simulink model "Model_plane1_new"  (R2024a)
settings: Solver=FixedStepAuto  StartTime=0  StopTime=2000  FixedStep=1  RelTol=1e-3
model workspace (MAT data in the model file):
  Alfa = [-2 4 10 16]
  Alfa_RUD = 0.55
  Alfa_table = [-4 0 5 10 20]
  Alfa_y = [-4 6 8 9 10 12 14]
  Cxa_table = [0.03434  0.0358  0.04274; 0.02598  0.0252  0.0262; 0.04151  0.0505  0.0883; 0.122  0.1649  0.2341; 0.502  0.538  0.666]
  Cy_DB = [0.01242 0.01286 0.01457]
  Cy_fi = [0.00623 0.00643 0.00626]
  Cya = [-0.276  -0.33  -0.39; 0.859  0.991  0.82; 1.085  1.211  1.1; 1.2  1.275  1.031; 1.296  1.29  1.018; 1.45  1.178  1.043; 1.461  1.163  1.081]
  Del_B = -5
  H = [339 3256 4060 8000 12000]
  H_table = [0 2000 4000 6000 8000 10000]
  I = [1000 1000 4500000]
  K_H = -0.3
  K_p = 0.3
  K_w = 1.5
  M_C = [0.4 0.6 0.82]
  M_mz = [0.2 0.4 0.6 0.8]
  M_mz2 = [0.4 0.7 0.85]
  M_table = [0.4 0.7 0.82]
  M_y = [0.4 0.7 0.82]
  P = [50000 40000 32000 25600 20480]
  Psi0 = 0
  Skr = 131
  Teta0 = 0
  V0 = 135
  a_table = [340.3 339.5 338.8 338 337.2 336.4]
  ba = 3.466
  fi = 0
  fi_P = 2
  g = 9.81
  lz = 4500000
  mla = 60000
  mz_DB = [-0.035 -0.0358 -0.037 -0.0377]
  mz_alfa = [-0.0282 -0.0282 -0.0289 -0.0404]
  mz_alfa2 = [-8.163  -8.762  -9.714; -8.163  -8.762  -9.583; -7.975  -7.991  -7.868; -6.514  -6.413  -6.732]
  mz_fi = [-0.0695 -0.0714 -0.0739 -0.0832]
  mz_omz = [-23.768  -25.3  -28.284; -23.768  -25.3  -27.903; -23.222  -22.6  -23.32; -18.967  -18.52  -19.601]
  n_dvig = 2
  out = Simulink.SimulationOutput
  out.Data.tout = [0 1.67688873362e-06 9.33181354111e-06 4.76064375786e-05 0.000238979557766 0.0011958451587 0.00598017316339 0.0291858115735 0.107609227908 0.294605508218 0.534390352194 0.619831316604 ... (6422 elements, 6422x1)]
  out.Metadata = Simulink.SimulationMetadata
  out.Metadata.ModelInfo.ModelName = 'Model_plane2'
  out.Metadata.ModelInfo.ModelVersion = '1.11'
  out.Metadata.ModelInfo.ModelFilePath = 'C:\Users\Анастасия\Универ\Mathlab\Модель самолёта\Model_plane2.slx'
  out.Metadata.ModelInfo.UserID = 'Анастасия'
  out.Metadata.ModelInfo.MachineName = 'DESKTOP-OE36224'
  out.Metadata.ModelInfo.Platform = 'PCWIN64'
  out.Metadata.ModelInfo.ModelStructuralChecksum = [329193822; 1830100004; 2373400892; 4162968501]
  out.Metadata.ModelInfo.SimulationMode = 'normal'
  out.Metadata.ModelInfo.StartTime = 0
  out.Metadata.ModelInfo.StopTime = 100
  out.Metadata.ModelInfo.SolverInfo.Type = 'Variable-Step'
  out.Metadata.ModelInfo.SolverInfo.Solver = 'ode45'
  out.Metadata.ModelInfo.SolverInfo.MaxStepSize = 2
  out.Metadata.ModelInfo.SimulinkVersion.Name = 'Simulink'
  out.Metadata.ModelInfo.SimulinkVersion.Version = '24.1'
  out.Metadata.ModelInfo.SimulinkVersion.Release = '(R2024a)'
  out.Metadata.ModelInfo.SimulinkVersion.Date = '19-Nov-2023'
  out.Metadata.ModelInfo.LoggingInfo.LoggingToFile = 'off'
  out.Metadata.TimingInfo.WallClockTimestampStart = '2025-02-14 11:01:22'
  out.Metadata.TimingInfo.WallClockTimestampStop = '2025-02-14 11:01:24'
  out.Metadata.TimingInfo.InitializationElapsedWallTime = 1.1990057
  out.Metadata.TimingInfo.ExecutionElapsedWallTime = 1.0786509
  out.Metadata.TimingInfo.TerminationElapsedWallTime = 0.0112241
  out.Metadata.TimingInfo.TotalElapsedWallTime = 2.2888807
  out.Metadata.TimingInfo.ProfilerData = 'Profiler is not enabled'
  out.Metadata.ExecutionInfo.StopEvent = 'ReachedStopTime'
  out.Metadata.ExecutionInfo.StopEventSource = []
  out.Metadata.ExecutionInfo.StopEventDescription = 'Reached stop time of 100'
  out.Metadata.ExecutionInfo.ErrorDiagnostic = []
  out.Metadata.ExecutionInfo.WarningDiagnostics.Diagnostic = MSLDiagnostic
  out.Metadata.ExecutionInfo.WarningDiagnostics.Diagnostic.identifier = 'Simulink:blocks:DivideByZero'
  out.Metadata.ExecutionInfo.WarningDiagnostics.Diagnostic.message = 'Division by zero in ''<a href="matlab:open_and_hilite_hyperlink (''Model_plane2/Уравнения продольного движения в связанной системе координат/Блок расчёта угла атаки Alfa/Divide'',''error'')">Model_plane2/Уравнения продольного движения в связанной системе координат/Блок расчёта угла атаки Alfa/Divide</a>'''
  out.Metadata.ExecutionInfo.WarningDiagnostics.Diagnostic.paths = {'Model_plane2/Уравнения продольного движения в связанной системе координат/Блок расчёта угла атаки Alfa/Divide'}
  out.Metadata.ExecutionInfo.WarningDiagnostics.Diagnostic.arguments = {'Model_plane2/Уравнения продольного движения в связанной системе координат/Блок расчёта угла атаки Alfa/Divide'}
  out.Metadata.ExecutionInfo.WarningDiagnostics.Diagnostic.stack = struct([])
  out.Metadata.ExecutionInfo.WarningDiagnostics.Diagnostic.actionProp = '22 serialization::archive 19 0 0 0  0 1 0 0 1 1 0 0 0 0 0 1 47 SL_SERVICES:utils:EMBEDDED____ACTION____WRAPPER 2 2 0 0 183 0 109 97 116 108 97 98 58 83 105 109 117 108 105 110 107 46 83 117 112 112 114 101 115 115 101 100 68 105 97 103 110 111 115 116 105 99 40 123 39 77 111 100 101 108 95 112 108 97 110 101 50 47 1059 1088 1072 1074 1085 1077 1085 1080 1103 32 1087 1088 1086 1076 1086 1083 1100 1085 1086 1075 1086 32 1076 1074 1080 1078 1077 1085 1080 1103 32 1074 32 1089 1074 1103 1079 1072 1085 1085 1086 1081 32 1089 1080 1089 1090 1077 1084 1077 32 1082 1086 1086 1088 1076 1080 1085 1072 1090 47 1041 1083 1086 1082 32 1088 1072 1089 1095 1105 1090 1072 32 1091 1075 1083 1072 32 1072 1090 1072 1082 1080 32 65 108 102 97 47 68 105 118 105 100 101 39 125 44 39 83 105 109 117 108 105 110 107 58 98 108 111 99 107 115 58 68 105 118 105 100 101 66 121 90 101 114 111 39 41 59 2 0 0 1 6 0 0 0 0 0  1 0 0 0 0'
  out.Metadata.ExecutionInfo.WarningDiagnostics.Diagnostic.metaDataProp.UI = []
  out.Metadata.ExecutionInfo.WarningDiagnostics.Diagnostic.metaDataProp.STAGE = []
  out.Metadata.ExecutionInfo.WarningDiagnostics.Diagnostic.metaDataProp.CATEGORY = []
  out.Metadata.ExecutionInfo.WarningDiagnostics.Diagnostic.metaDataProp.COMPONENT = []
  out.Metadata.ExecutionInfo.WarningDiagnostics.Diagnostic.metaDataProp.MDL_NAME = []
  out.Metadata.ExecutionInfo.WarningDiagnostics.Diagnostic.metaDataProp.ACTION = '22 serialization::archive 19 0 0 0  0 1 0 0 1 1 0 0 0 0 0 1 47 SL_SERVICES:utils:EMBEDDED____ACTION____WRAPPER 2 2 0 0 183 0 109 97 116 108 97 98 58 83 105 109 117 108 105 110 107 46 83 117 112 112 114 101 115 115 101 100 68 105 97 103 110 111 115 116 105 99 40 123 39 77 111 100 101 108 95 112 108 97 110 101 50 47 1059 1088 1072 1074 1085 1077 1085 1080 1103 32 1087 1088 1086 1076 1086 1083 1100 1085 1086 1075 1086 32 1076 1074 1080 1078 1077 1085 1080 1103 32 1074 32 1089 1074 1103 1079 1072 1085 1085 1086 1081 32 1089 1080 1089 1090 1077 1084 1077 32 1082 1086 1086 1088 1076 1080 1085 1072 1090 47 1041 1083 1086 1082 32 1088 1072 1089 1095 1105 1090 1072 32 1091 1075 1083 1072 32 1072 1090 1072 1082 1080 32 65 108 102 97 47 68 105 118 105 100 101 39 125 44 39 83 105 109 117 108 105 110 107 58 98 108 111 99 107 115 58 68 105 118 105 100 101 66 121 90 101 114 111 39 41 59 2 0 0 1 6 0 0 0 0 0  1 0 0 0 0'
  out.Metadata.ExecutionInfo.WarningDiagnostics.Diagnostic.metaDataProp.DOC = []
  out.Metadata.ExecutionInfo.WarningDiagnostics.Diagnostic.metaDataProp.SUB_CATEGORY = []
  out.Metadata.ExecutionInfo.WarningDiagnostics.Diagnostic.metaDataProp.MSTACK_PRESERVE = []
  out.Metadata.ExecutionInfo.WarningDiagnostics.Diagnostic.metaDataProp.DOUBLE_ARGS = []
  out.Metadata.ExecutionInfo.WarningDiagnostics.Diagnostic.metaDataProp.USER_DATA = []
  out.Metadata.ExecutionInfo.WarningDiagnostics.Diagnostic.priority = 2
  out.Metadata.ExecutionInfo.WarningDiagnostics.SimulationPhase = 'Execution'
  out.Metadata.ExecutionInfo.WarningDiagnostics.SimulationTime = 0
  out.Metadata.AppInfo = struct()
  pitch = 1
  pitch0 = 0
  q_table = [1.225 1.0065 0.8194 0.6601 0.5258 0.4135]
  roll0 = 0
  wx0 = 0
  wy0 = 0
  wz0 = 0
  x0 = 0
  xy = [240000 6200]
  y0 = 5000
  yaw0 = 0
  z0 = 0
settings Model: Creator=Анастасия  LastModifiedBy=Анастасия
settings SolverCC: MaxConsecutiveMinStep=5
settings DebuggingCC: UnderSpecifiedDimensionMsg=warning

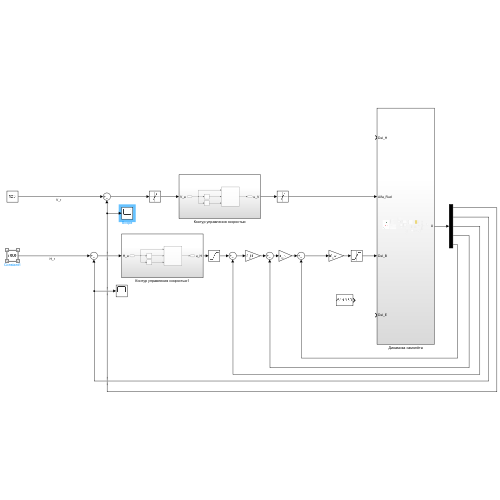
[thumbnail: Simulink's stored preview of the top-level diagram]
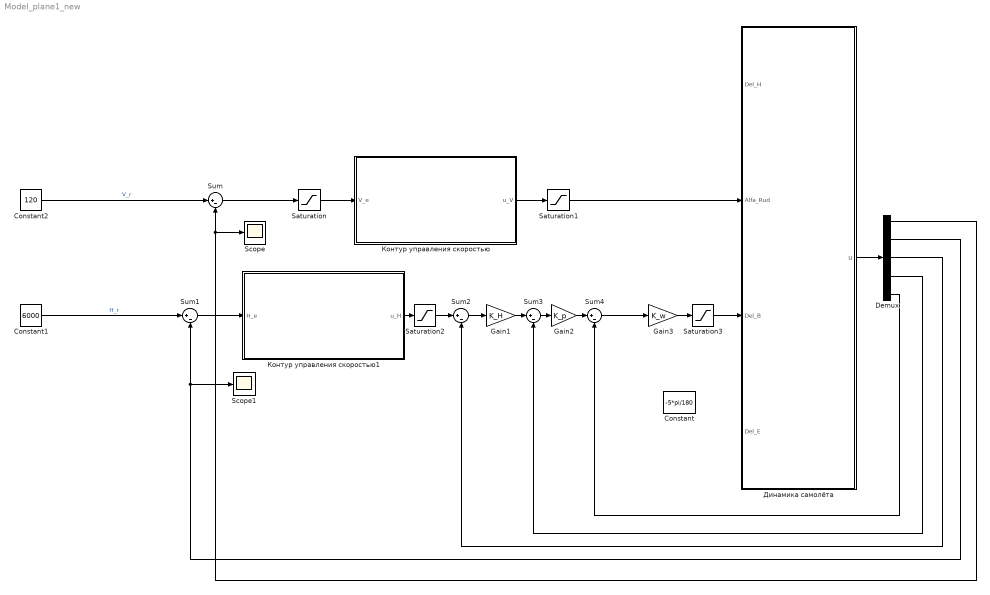
== system Model_plane1_new ==
  Constant : Constant  Value=-5*pi/180
  Constant1 : Constant  Value=6000
  Constant2 : Constant  Value=120
  Demux : Demux  Outputs=5
  Gain1 : Gain  Gain=K_H
  Gain2 : Gain  Gain=K_p
  Gain3 : Gain  Gain=K_w
  Saturation : Saturate  UpperLimit=300  LowerLimit=-300
  Saturation1 : Saturate  UpperLimit=300  LowerLimit=0
  Saturation2 : Saturate  UpperLimit=10  LowerLimit=-10
  Saturation3 : Saturate  UpperLimit=25*pi/180  LowerLimit=-35*pi/180
  Scope : Scope
  Scope1 : Scope
  Sum{,1..4} (5 alike) : Sum  Inputs=|+-
  Динамика самолёта : Subsystem
  Контур управления скоростью : Subsystem
  Контур управления скоростью1 : Subsystem
  wires:
  Constant2/1 -> Sum/1  "V_r"
  Sum/1 -> Saturation/1
  Saturation/1 -> Контур управления скоростью/1(V_e)
  Контур управления скоростью/1(u_V) -> Saturation1/1
  Динамика самолёта/1(U) -> Demux/1
  Demux/1 -> Scope/1, Sum/2
  Constant1/1 -> Sum1/1  "H_r"
  Demux/2 -> Scope1/1, Sum1/2
  Sum1/1 -> Контур управления скоростью1/1(H_e)
  Контур управления скоростью1/1(u_H) -> Saturation2/1
  Saturation2/1 -> Sum2/1
  Sum2/1 -> Gain1/1
  Gain1/1 -> Sum3/1
  Sum3/1 -> Gain2/1
  Gain2/1 -> Sum4/1
  Sum4/1 -> Gain3/1
  Gain3/1 -> Saturation3/1
  Demux/3 -> Sum2/2
  Demux/4 -> Sum3/2
  Demux/5 -> Sum4/2
  Saturation1/1 -> Динамика самолёта/2(Alfa_Rud)
  Saturation3/1 -> Динамика самолёта/3(Del_B)

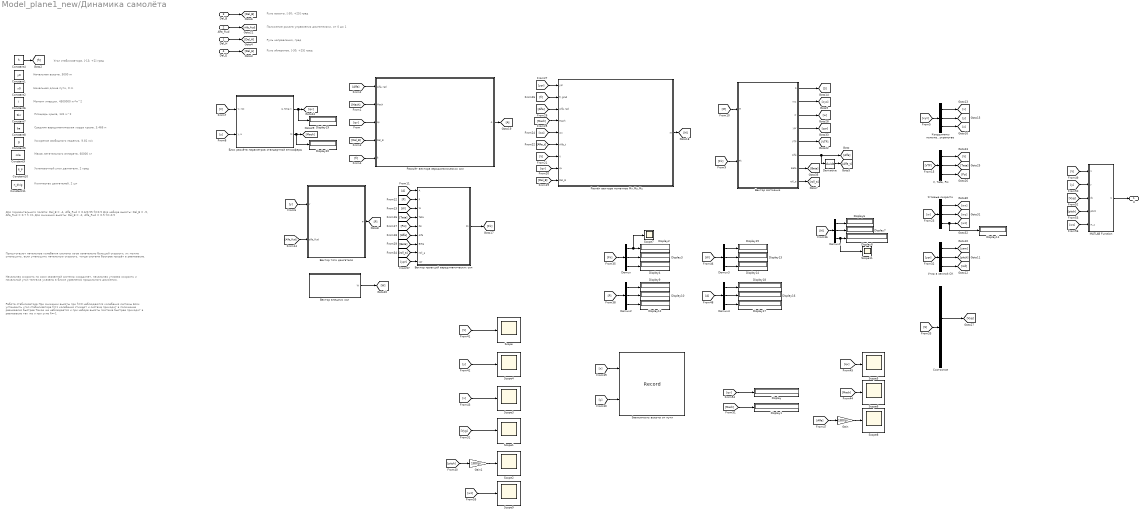
== system Model_plane1_new/Динамика самолёта ==
  note: Руль высоты, [-30; +25] град
  note: Начальная скорость по осям связанной системы координат, начальная угловая скорость и начальный угол тангажа указаны в блоке уравнения продольного движения.
  note: Количество двигателей, 2 шт
  note: Присутствуют начальные колебания системы из-за изначально большой скорости, их можно уменьшить, если уменьшить начальную скорость, тогда система быстрее придёт в равновесие.
  note: Установочный угол двигателя, 2 град
  note: Ускорение свободного падения, 9.81 м/c
  note: Масса летательного аппарата, 60000 кг
  note: Положение рычага управления двигателями, от 0 до 1
  note: Для горизонтального полёта:
      | Del_B = -4, Alfa_Rud = 0.6/0.55 fi=0.5
      | Для набора высоты:
      | Del_B = -5, Alfa_Rud = 0.7 fi =1
      | Для снижения высоты:
      | Del_B = -2, Alfa_Rud = 0.5 fi=-0.5
  note: Начальная длина пути, 0 m
  note: Работа стабилизатора
      | При снижении высоты при fi=0 наблюдаются колебания системы
      | Если установить угол стабилизатора fi=1 колебания стихают и систама приходит в положение равновесия быстрее
      | Такое же наблюдается и при наборе высоты (система быстрее приходит в равновесие так же и при угле fi=-1
  note: Средняя аэродинамическая хорда крыла, 3.466 м
  note: Площадь крыла, 131 м^2
  note: Начальная высота, 5000 m
  note: Момент инерции, 4500000 кг*м^2
  note: Угол стабилизатора, [-13; +2] град
  note: Руль направления, град
  note: Руль эйлеронов, [-30; +25] град
  Del_H : Inport
  Alfa_Rud : Inport  Port=2
  Del_B : Inport  Port=3
  Del_E : Inport  Port=4
  Constant1 : Constant  Value=y0
  Constant10 : Constant  Value=fi_P
  Constant11 : Constant  Value=n_dvig
  Constant2 : Constant  Value=x0
  Constant4 : Constant  Value=fi
  Constant5 : Constant  Value=g
  Constant6 : Constant  Value=I
  Constant7 : Constant  Value=Skr
  Constant8 : Constant  Value=ba
  Constant9 : Constant  Value=mla
  Demux{,1..4} (5 alike) : Demux  Outputs=3
  Derivative : Derivative
  Display{,1..4,6..20} (20 alike) : Display
  From11 : From
  From48 : From
  Gain : Gain  Gain=180/pi
  Gain1 : Gain  Gain=180/pi
  Goto19 : Goto
  MATLAB Function : MATLAB Function  TreatAsAtomicUnit=on
  Scope{,1..9,11} (11 alike) : Scope
  "V, Teta, Psi" : Demux  Outputs=3
  Блок расчёта параметров стандартной атмосферы : Subsystem
  Вектор внешних сил : Subsystem
  Вектор проекций аэродинамических сил : Subsystem
  Вектор состояния : Subsystem
  Вектор тяги двигателя : Subsystem
  Зависимость высоты от пути : Record  FileSettingsInternal="{\"entries\":[{\"content\":{\"excelSettings\":{\"content\":{},\"type\":\"Streamout.ExcelSettings\"}},\"type\":\"Streamout.FileSettingStorage\",\"uuid\":\"\"}],\"packageUris\":[\"http:\\/\\/schema.mathworks.com\\/mf0\\/streamout_blocks\\/R2020a\"],\"version\":\"1.0\"}"  Layout=[1 1]  SignalsInternal="{\"entries\":[{\"content\":{\"signals\":[{\"content\":{\"blockPath\":[],\"dimensions\":[1],\"domain\":\"\",\"lineColor\":\"#a2142f\",\"plots\":[ 1 ],\"port\":1,\"sid\":[\"\"],\"signalID\":1,\"signalName\":\"From39\"},\"type\":\"RecordBlkView.Signal\",\"uuid\":\"\"},{\"content\":{\"blockPath\":[],\"dimensions\":[1],\"domain\":\"\",\"lineColor\":\"#139fff\",\"plots\":[ 1 ],\"port\":2,\"sid\":[\"\"],\"signalID\":2,\"signalName\":\"From30\"},\"type\":\"RecordBlkView.Signal\",\"uuid\":\"\"}]},\"type\":\"RecordBlkView.InputSignals\",\"uuid\":\"\"}],\"packageUris\":[\"http:\\/\\/schema.mathworks.com\\/mf0\\/streamout_blocks\\/R2020a\"],\"version\":\"1.0\"}"  VisualizationBindings="{\"xyplotplugin\":{\"info\":[{\"series\":[{\"bindingParametersList\":[{\"parameter\":\"X-Axis\",\"signalID\":1,\"signalName\":\"From39\"},{\"parameter\":\"Y-Axis\",\"signalID\":2,\"signalName\":\"From30\"}],\"seriesID\":0}],\"subplotID\":1}]}}"  CompatibilityTag=XY  st=-1
  Координаты положения в пространстве : Demux  Outputs=3
  Рассчёт вектора аэродинамических сил : Subsystem
  Расчёт вектора мометнов Mx,My,Mz : Subsystem
  Состояние : Demux  Outputs=12
  Угловые скорости : Demux  Outputs=3
  Углы в земной СК : Demux  Outputs=3
  U : Outport
  wires:
  Constant4/1 -> [fi]
  [V] -> Блок расчёта параметров стандартной атмосферы/1("V, м/с")
  [y] -> Блок расчёта параметров стандартной атмосферы/2("y, м")
  Блок расчёта параметров стандартной атмосферы/2(М) -> Display20/1, [Mach]
  Блок расчёта параметров стандартной атмосферы/1("q, Н/кв.м") -> Display19/1, [qv]
  Вектор состояния/6(Alfa) -> Derivative/1, [Alfa]
  Derivative/1 -> [Alfa_t]
  [qv] -> Рассчёт вектора аэродинамических сил/3(qv)
  [Mach] -> Рассчёт вектора аэродинамических сил/2(Mach)
  [Alfa] -> Рассчёт вектора аэродинамических сил/1("Alfa, rad")
  [Del_B] -> Рассчёт вектора аэродинамических сил/4(Del_B)
  Del_B/1 -> [Del_B]
  [fi] -> Рассчёт вектора аэродинамических сил/5(fi)
  Вектор тяги двигателя/1(P) -> [P]
  Вектор состояния/2(xyz) -> [xyz]
  [xyz] -> Координаты положения в пространстве/1
  Координаты положения в пространстве/1 -> [x]
  Координаты положения в пространстве/2 -> [y]
  Координаты положения в пространстве/3 -> [z]
  [y] -> Вектор тяги двигателя/1(y)
  Вектор проекций аэродинамических сил/1(Fk) -> [Fk]
  [Fk] -> Вектор состояния/2(Fk)
  Расчёт вектора мометнов Mx,My,Mz/1(M) -> [M]
  Рассчёт вектора аэродинамических сил/1(A) -> Goto19/1
  From11/1 -> Вектор проекций аэродинамических сил/1(A)
  Вектор внешних сил/1(W) -> [W]
  [P] -> Вектор проекций аэродинамических сил/2(P)
  [W] -> Вектор проекций аэродинамических сил/3(W)
  Alfa_Rud/1 -> [Alfa_Rud]
  [Alfa_Rud] -> Вектор тяги двигателя/2(alfa_Rud)
  Вектор состояния/5(VTP) -> [VTP]
  [VTP] -> "V, Teta, Psi"/1
  "V, Teta, Psi"/3 -> [Psi]
  "V, Teta, Psi"/2 -> [Teta]
  "V, Teta, Psi"/1 -> [V]
  [Psi] -> Вектор проекций аэродинамических сил/5(Psi)
  [Teta] -> Вектор проекций аэродинамических сил/4(Teta)
  [Alfa] -> Вектор проекций аэродинамических сил/6(Alfa)
  [Del_B] -> Расчёт вектора мометнов Mx,My,Mz/9(Del_B)
  [qv] -> Расчёт вектора мометнов Mx,My,Mz/8(qv)
  [V] -> Расчёт вектора мометнов Mx,My,Mz/7(V)
  [Alfa_t] -> Расчёт вектора мометнов Mx,My,Mz/6(Alfa_t)
  Вектор состояния/3(w) -> [w]
  Угловые скорости/3 -> Display11/1, [wz]
  Угловые скорости/2 -> [wy]
  Угловые скорости/1 -> [wx]
  [w] -> Угловые скорости/1
  [wz] -> Расчёт вектора мометнов Mx,My,Mz/5(wz)
  [Mach] -> Расчёт вектора мометнов Mx,My,Mz/4(Mach)
  [fi] -> Расчёт вектора мометнов Mx,My,Mz/2("fi, grad")
  Вектор состояния/4(ypr) -> [ypr]
  [ypr] -> Расчёт вектора мометнов Mx,My,Mz/1(ypr)
  [Alfa] -> Расчёт вектора мометнов Mx,My,Mz/3("Alfa, rad")
  Del_H/1 -> [Del_H]
  Del_E/1 -> [Del_E]
  [wz] -> Scope9/1
  [V] -> Scope/1
  [Mach] -> Display1/1
  [x] -> Зависимость высоты от пути/1
  [qv] -> Scope5/1
  [Alfa] -> Gain/1
  Gain1/1 -> Scope2/1
  [qv] -> Display/1
  [Vyg] -> Scope1/1
  [x] -> Scope3/1
  [Mach] -> Scope6/1
  [pitch] -> Gain1/1
  [y] -> Scope4/1
  [y] -> Зависимость высоты от пути/2
  [ypr] -> Углы в земной СК/1
  Вектор состояния/1(S) -> [S]
  Состояние/5 -> [Vyg]
  Вектор состояния/7(Beta) -> [Beta]
  [M] -> Вектор состояния/1(M)
  Углы в земной СК/1 -> [yaw]
  Углы в земной СК/2 -> [pitch]
  Углы в земной СК/3 -> [roll]
  [S] -> Состояние/1
  [Fk] -> Demux/1
  Demux/1 -> Scope7/1, Display2/1
  Demux/2 -> Display3/1
  Demux/3 -> Display4/1
  [M] -> Demux1/1
  Demux1/1 -> Display6/1
  Demux1/2 -> Display7/1
  Demux1/3 -> Scope11/1, Display8/1
  Вектор состояния/8(roll_a) -> [roll_a]
  Demux2/2 -> Display10/1
  Demux2/3 -> Display12/1
  Demux2/1 -> Display9/1
  [P] -> Demux2/1
  Demux3/3 -> Display14/1
  Demux3/1 -> Display15/1
  Demux3/2 -> Display13/1
  [W] -> Demux3/1
  Demux4/3 -> Display17/1
  Demux4/1 -> Display18/1
  Demux4/2 -> Display16/1
  From48/1 -> Demux4/1
  [Beta] -> Вектор проекций аэродинамических сил/7(Beta)
  [roll_a] -> Вектор проекций аэродинамических сил/8(roll_a)
  Gain/1 -> Scope8/1
  [V] -> MATLAB Function/1(V)
  MATLAB Function/1(U) -> U/1
  [wz] -> MATLAB Function/5(w_z)
  [pitch] -> MATLAB Function/4(pitch)
  [Vyg] -> MATLAB Function/3(dy)
  [y] -> MATLAB Function/2(y)
  [ypr] -> Вектор проекций аэродинамических сил/9(ypr)

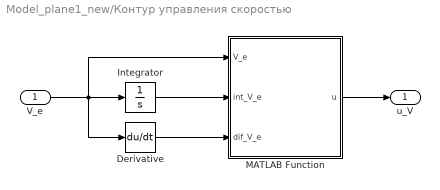
== system Model_plane1_new/Контур управления скоростью ==
  V_e : Inport
  Derivative : Derivative
  Integrator : Integrator
  MATLAB Function : MATLAB Function  TreatAsAtomicUnit=on
  u_V : Outport
  wires:
  V_e/1 -> Derivative/1, MATLAB Function/1(V_e), Integrator/1
  MATLAB Function/1(u) -> u_V/1
  Integrator/1 -> MATLAB Function/2(int_V_e)
  Derivative/1 -> MATLAB Function/3(dif_V_e)

== system Model_plane1_new/Контур управления скоростью1 ==
  H_e : Inport
  Derivative : Derivative
  Integrator : Integrator
  MATLAB Function : MATLAB Function  TreatAsAtomicUnit=on
  u_H : Outport
  wires:
  H_e/1 -> Derivative/1, MATLAB Function/1(H_e), Integrator/1
  MATLAB Function/1(u) -> u_H/1
  Integrator/1 -> MATLAB Function/2(int_H_e)
  Derivative/1 -> MATLAB Function/3(dif_H_e)

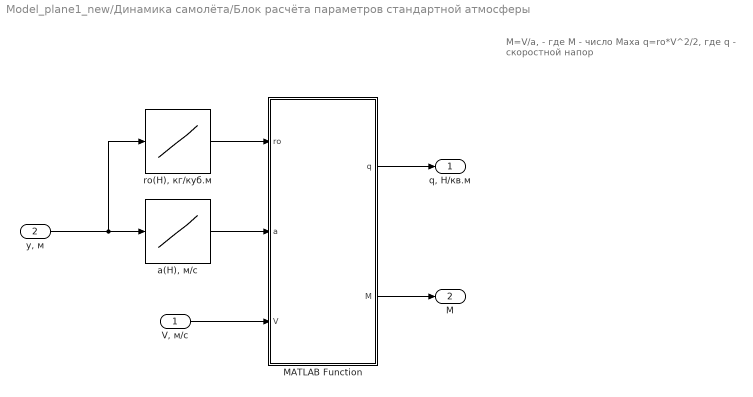
== system Model_plane1_new/Динамика самолёта/Блок расчёта параметров стандартной атмосферы ==
  note: M=V/a, - где М - число Маха
      | q=ro*V^2/2, где q - скоростной напор
  "V, м/с" : Inport
  "y, м" : Inport  Port=2
  MATLAB Function : MATLAB Function  TreatAsAtomicUnit=on
  "a(H), м/с" : Lookup_n-D  NumberOfTableDimensions=1  BreakpointsForDimension1=H_table  Table=a_table  InternalRulePriority=Speed  RndMeth=Simplest
  "ro(H), кг/куб.м" : Lookup_n-D  NumberOfTableDimensions=1  BreakpointsForDimension1=H_table  Table=q_table  InternalRulePriority=Speed  RndMeth=Simplest
  "q, Н/кв.м" : Outport
  М : Outport  Port=2
  wires:
  "y, м"/1 -> "ro(H), кг/куб.м"/1, "a(H), м/с"/1
  "ro(H), кг/куб.м"/1 -> MATLAB Function/1(ro)
  "a(H), м/с"/1 -> MATLAB Function/2(a)
  MATLAB Function/1(q) -> "q, Н/кв.м"/1
  MATLAB Function/2(M) -> М/1
  "V, м/с"/1 -> MATLAB Function/3(V)

== system Model_plane1_new/Динамика самолёта/Вектор внешних сил ==
  Constant : Constant  Value=mla
  Constant1 : Constant  Value=g
  MATLAB Function : MATLAB Function  TreatAsAtomicUnit=on
  W : Outport
  wires:
  Constant/1 -> MATLAB Function/1(mla)
  MATLAB Function/1(W) -> W/1
  Constant1/1 -> MATLAB Function/2(g)

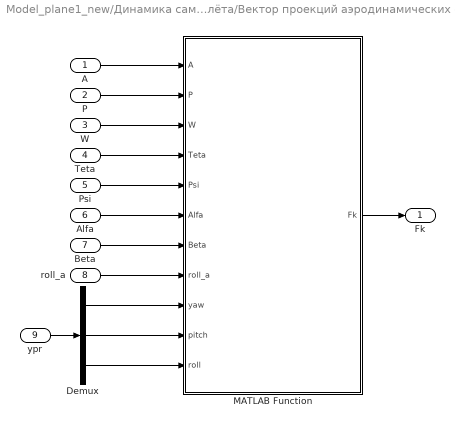
== system Model_plane1_new/Динамика самолёта/Вектор проекций аэродинамических сил ==
  A : Inport
  P : Inport  Port=2
  W : Inport  Port=3
  Teta : Inport  Port=4
  Psi : Inport  Port=5
  Alfa : Inport  Port=6
  Beta : Inport  Port=7
  roll_a : Inport  Port=8
  ypr : Inport  Port=9
  Demux : Demux  Outputs=3
  MATLAB Function : MATLAB Function  TreatAsAtomicUnit=on
  Fk : Outport
  wires:
  MATLAB Function/1(Fk) -> Fk/1
  A/1 -> MATLAB Function/1(A)
  P/1 -> MATLAB Function/2(P)
  W/1 -> MATLAB Function/3(W)
  Psi/1 -> MATLAB Function/5(Psi)
  Teta/1 -> MATLAB Function/4(Teta)
  Alfa/1 -> MATLAB Function/6(Alfa)
  Beta/1 -> MATLAB Function/7(Beta)
  roll_a/1 -> MATLAB Function/8(roll_a)
  ypr/1 -> Demux/1
  Demux/1 -> MATLAB Function/9(yaw)
  Demux/2 -> MATLAB Function/10(pitch)
  Demux/3 -> MATLAB Function/11(roll)

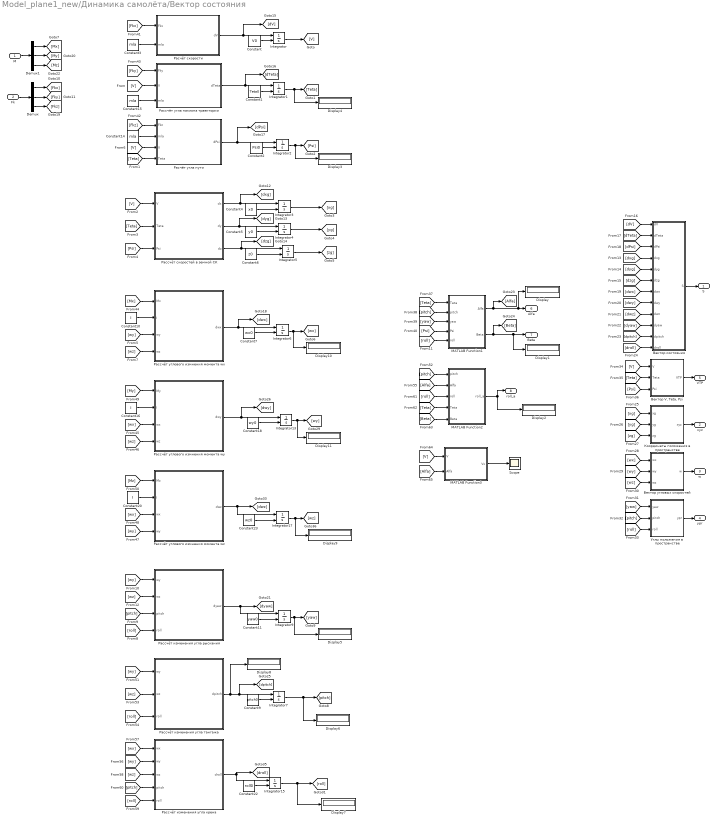
== system Model_plane1_new/Динамика самолёта/Вектор состояния ==
  M : Inport
  Fk : Inport  Port=2
  Constant : Constant  Value=V0
  Constant1 : Constant  Value=Teta0
  Constant10 : Constant  Value=I
  Constant11 : Constant  Value=yaw0
  Constant14 : Constant  Value=mla
  Constant15 : Constant  Value=mla
  Constant16 : Constant  Value=I
  Constant18 : Constant  Value=wy0
  Constant2 : Constant  Value=Psi0
  Constant20 : Constant  Value=I
  Constant22 : Constant  Value=roll0
  Constant23 : Constant  Value=wz0
  Constant3 : Constant  Value=mla
  Constant4 : Constant  Value=x0
  Constant5 : Constant  Value=y0
  Constant6 : Constant  Value=z0
  Constant7 : Constant  Value=wx0
  Constant9 : Constant  Value=pitch0
  Demux : Demux  Outputs=3
  Demux1 : Demux  Outputs=3
  Display{,1..11} (12 alike) : Display
  Integrator{,1..7,9,13,15,17} (12 alike) : Integrator  InitialConditionSource=external
  MATLAB Function1 : MATLAB Function  TreatAsAtomicUnit=on
  MATLAB Function2 : MATLAB Function  TreatAsAtomicUnit=on
  MATLAB Function3 : MATLAB Function  TreatAsAtomicUnit=on
  Scope : Scope
  "Вектор V, Teta, Psi" : MATLAB Function  TreatAsAtomicUnit=on
  Вектор состояния : MATLAB Function  TreatAsAtomicUnit=on
  Вектор угловых скоростей : MATLAB Function  TreatAsAtomicUnit=on
  Координаты положения в пространстве : MATLAB Function  TreatAsAtomicUnit=on
  Рассчёт изменения угла крена : MATLAB Function  TreatAsAtomicUnit=on
  Рассчёт изменения угла рыскания : MATLAB Function  TreatAsAtomicUnit=on
  Рассчёт изменения угла тангажа : MATLAB Function  TreatAsAtomicUnit=on
  Рассчёт скоростей в земной СК : MATLAB Function  TreatAsAtomicUnit=on
  Рассчёт угла наклона траектории : MATLAB Function  TreatAsAtomicUnit=on
  Рассчёт углового измнения момента wx : MATLAB Function  TreatAsAtomicUnit=on
  Рассчёт углового измнения момента wy : MATLAB Function  TreatAsAtomicUnit=on
  Рассчёт углового измнения момента wz : MATLAB Function  TreatAsAtomicUnit=on
  Расчёт скорости : MATLAB Function  TreatAsAtomicUnit=on
  Расчёт угла пути : MATLAB Function  TreatAsAtomicUnit=on
  Углы положения в пространстве : MATLAB Function  TreatAsAtomicUnit=on
  S : Outport
  xyz : Outport  Port=2
  w : Outport  Port=3
  ypr : Outport  Port=4
  VTP : Outport  Port=5
  Alfa : Outport  Port=6
  Beta : Outport  Port=7
  roll_a : Outport  Port=8
  wires:
  Рассчёт скоростей в земной СК/3(dz) -> [dzg], Integrator5/1
  Рассчёт скоростей в земной СК/2(dy) -> [dyg], Integrator4/1
  Рассчёт скоростей в земной СК/1(dx) -> [dxg], Integrator3/1
  [V] -> Рассчёт скоростей в земной СК/1(V)
  [Teta] -> Рассчёт скоростей в земной СК/2(Teta)
  [Psi] -> Рассчёт скоростей в земной СК/3(Psi)
  Integrator3/1 -> [xg]
  Integrator5/1 -> [zg]
  Integrator4/1 -> [yg]
  Constant4/1 -> Integrator3/2
  Constant6/1 -> Integrator5/2
  Constant5/1 -> Integrator4/2
  Рассчёт углового измнения момента wx/1(dwx) -> [dwx], Integrator6/1
  Constant7/1 -> Integrator6/2
  Integrator6/1 -> Display10/1, [wx]
  [wz] -> Рассчёт углового измнения момента wx/4(wz)
  [wy] -> Рассчёт углового измнения момента wx/3(wy)
  Constant10/1 -> Рассчёт углового измнения момента wx/2(I)
  Constant11/1 -> Integrator9/2
  Integrator9/1 -> Display5/1, [yaw]
  Рассчёт изменения угла рыскания/1(dyaw) -> [dyaw], Integrator9/1
  [roll] -> Рассчёт изменения угла рыскания/4(roll)
  [pitch] -> Рассчёт изменения угла рыскания/3(pitch)
  [wy] -> Рассчёт изменения угла рыскания/1(wy)
  [wz] -> Рассчёт изменения угла рыскания/2(wz)
  [dV] -> Вектор состояния/1(dV)
  [dTeta] -> Вектор состояния/2(dTeta)
  [dPsi] -> Вектор состояния/3(dPsi)
  [dxg] -> Вектор состояния/4(dxg)
  [dyg] -> Вектор состояния/5(dyg)
  [dzg] -> Вектор состояния/6(dzg)
  [dwx] -> Вектор состояния/7(dwx)
  [dwy] -> Вектор состояния/8(dwy)
  [dwz] -> Вектор состояния/9(dwz)
  [dyaw] -> Вектор состояния/10(dyaw)
  [dpitch] -> Вектор состояния/11(dpitch)
  [droll] -> Вектор состояния/12(droll)
  Вектор состояния/1(S) -> S/1
  [xg] -> Координаты положения в пространстве/1(xg)
  [yg] -> Координаты положения в пространстве/2(yg)
  [zg] -> Координаты положения в пространстве/3(zg)
  Координаты положения в пространстве/1(xyz) -> xyz/1
  [wx] -> Вектор угловых скоростей/1(wx)
  Вектор угловых скоростей/1(w) -> w/1
  [wz] -> Вектор угловых скоростей/3(wz)
  [wy] -> Вектор угловых скоростей/2(wy)
  [yaw] -> Углы положения в пространстве/1(yaw)
  Углы положения в пространстве/1(ypr) -> ypr/1
  [roll] -> Углы положения в пространстве/3(roll)
  [pitch] -> Углы положения в пространстве/2(pitch)
  [V] -> "Вектор V, Teta, Psi"/1(V)
  "Вектор V, Teta, Psi"/1(VTP) -> VTP/1
  [Psi] -> "Вектор V, Teta, Psi"/3(Psi)
  [Teta] -> "Вектор V, Teta, Psi"/2(Teta)
  [Teta] -> MATLAB Function1/1(Teta)
  [pitch] -> MATLAB Function1/2(pitch)
  [yaw] -> MATLAB Function1/3(yaw)
  [Psi] -> MATLAB Function1/4(Psi)
  Integrator/1 -> [V]
  [Fkx] -> Расчёт скорости/1(Fkx)
  Constant14/1 -> Расчёт угла пути/2(mla)
  Constant2/1 -> Integrator2/2
  Constant/1 -> Integrator/2
  Расчёт скорости/1(dV) -> [dV], Integrator/1
  [Teta] -> Расчёт угла пути/4(Teta)
  Расчёт угла пути/1(dPsi) -> [dPsi], Integrator2/1
  [Fkz] -> Расчёт угла пути/1(Fkz)
  Integrator2/1 -> [Psi], Display3/1
  Constant3/1 -> Расчёт скорости/2(mla)
  Integrator1/1 -> [Teta], Display4/1
  Constant1/1 -> Integrator1/2
  Рассчёт угла наклона траектории/1(dTeta) -> Integrator1/1, [dTeta]
  [V] -> Рассчёт угла наклона траектории/2(V)
  [Fky] -> Рассчёт угла наклона траектории/1(Fky)
  Constant15/1 -> Рассчёт угла наклона траектории/3(mla)
  Рассчёт углового измнения момента wy/1(dwy) -> [dwy], Integrator13/1
  [wz] -> Рассчёт углового измнения момента wy/4(wz)
  [wx] -> Рассчёт углового измнения момента wy/3(wx)
  Integrator13/1 -> Display11/1, [wy]
  Constant18/1 -> Integrator13/2
  [wy] -> Рассчёт углового измнения момента wz/4(wy)
  Рассчёт углового измнения момента wz/1(dwz) -> Integrator17/1, [dwz]
  [wx] -> Рассчёт углового измнения момента wz/3(wx)
  Integrator17/1 -> Display9/1, [wz]
  Constant23/1 -> Integrator17/2
  Constant20/1 -> Рассчёт углового измнения момента wz/2(I)
  [V] -> Расчёт угла пути/3(V)
  M/1 -> Demux1/1
  [Mx] -> Рассчёт углового измнения момента wx/1(Mx)
  [My] -> Рассчёт углового измнения момента wy/1(My)
  [Mz] -> Рассчёт углового измнения момента wz/1(Mz)
  Рассчёт изменения угла тангажа/1(dpitch) -> Display8/1, [dpitch], Integrator7/1
  [wz] -> Рассчёт изменения угла тангажа/2(wz)
  [wy] -> Рассчёт изменения угла тангажа/1(wy)
  Integrator7/1 -> Display6/1, [pitch]
  Constant9/1 -> Integrator7/2
  [roll] -> Рассчёт изменения угла тангажа/3(roll)
  Constant22/1 -> Integrator15/2
  [pitch] -> Рассчёт изменения угла крена/4(pitch)
  Integrator15/1 -> Display7/1, [roll]
  Рассчёт изменения угла крена/1(droll) -> Integrator15/1, [droll]
  [wz] -> Рассчёт изменения угла крена/3(wz)
  [wy] -> Рассчёт изменения угла крена/2(wy)
  [wx] -> Рассчёт изменения угла крена/1(wx)
  [roll] -> Рассчёт изменения угла крена/5(roll)
  Fk/1 -> Demux/1
  Demux/1 -> [Fkx]
  Demux/2 -> [Fky]
  Demux/3 -> [Fkz]
  Demux1/1 -> [Mx]
  Demux1/2 -> [My]
  Demux1/3 -> [Mz]
  Constant16/1 -> Рассчёт углового измнения момента wy/2(I)
  MATLAB Function1/1(Alfa) -> Alfa/1, Display/1, [Alfa]
  MATLAB Function1/2(Beta) -> Display1/1, Beta/1, [Beta]
  MATLAB Function2/1(roll_a) -> Display2/1, roll_a/1
  [pitch] -> MATLAB Function2/1(pitch)
  [Alfa] -> MATLAB Function2/2(Alfa)
  [roll] -> MATLAB Function2/3(roll)
  [Teta] -> MATLAB Function2/4(Teta)
  [roll] -> MATLAB Function1/5(roll)
  [Beta] -> MATLAB Function2/5(Beta)
  [V] -> MATLAB Function3/1(V)
  [Alfa] -> MATLAB Function3/2(Alfa)
  MATLAB Function3/1(Vx) -> Scope/1

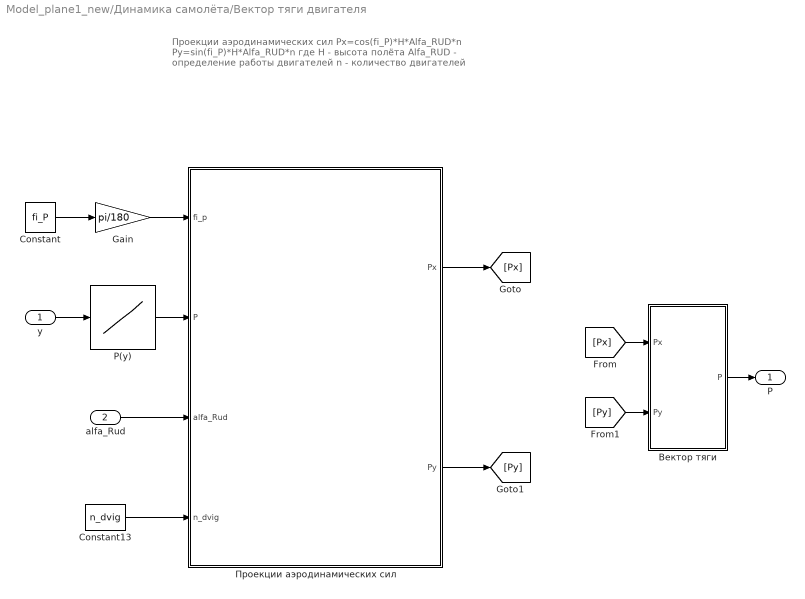
== system Model_plane1_new/Динамика самолёта/Вектор тяги двигателя ==
  note: Проекции аэродинамических сил
      | Px=cos(fi_P)*H*Alfa_RUD*n
      | Py=sin(fi_P)*H*Alfa_RUD*n
      | где Н - высота полёта
      | Alfa_RUD - определение работы двигателей
      | n - количество двигателей
  y : Inport
  alfa_Rud : Inport  Port=2
  Constant : Constant  Value=fi_P
  Constant13 : Constant  Value=n_dvig
  Gain : Gain  Gain=pi/180
  P(y) : Lookup_n-D  NumberOfTableDimensions=1  BreakpointsForDimension1=H  Table=P  InternalRulePriority=Speed  RndMeth=Simplest
  Вектор тяги : MATLAB Function  TreatAsAtomicUnit=on
  Проекции аэродинамических сил : MATLAB Function  TreatAsAtomicUnit=on
  P : Outport
  wires:
  P(y)/1 -> Проекции аэродинамических сил/2(P)
  Проекции аэродинамических сил/2(Py) -> [Py]
  alfa_Rud/1 -> Проекции аэродинамических сил/3(alfa_Rud)
  Проекции аэродинамических сил/1(Px) -> [Px]
  Constant/1 -> Gain/1
  y/1 -> P(y)/1
  Constant13/1 -> Проекции аэродинамических сил/4(n_dvig)
  [Px] -> Вектор тяги/1(Px)
  [Py] -> Вектор тяги/2(Py)
  Вектор тяги/1(P) -> P/1
  Gain/1 -> Проекции аэродинамических сил/1(fi_p)

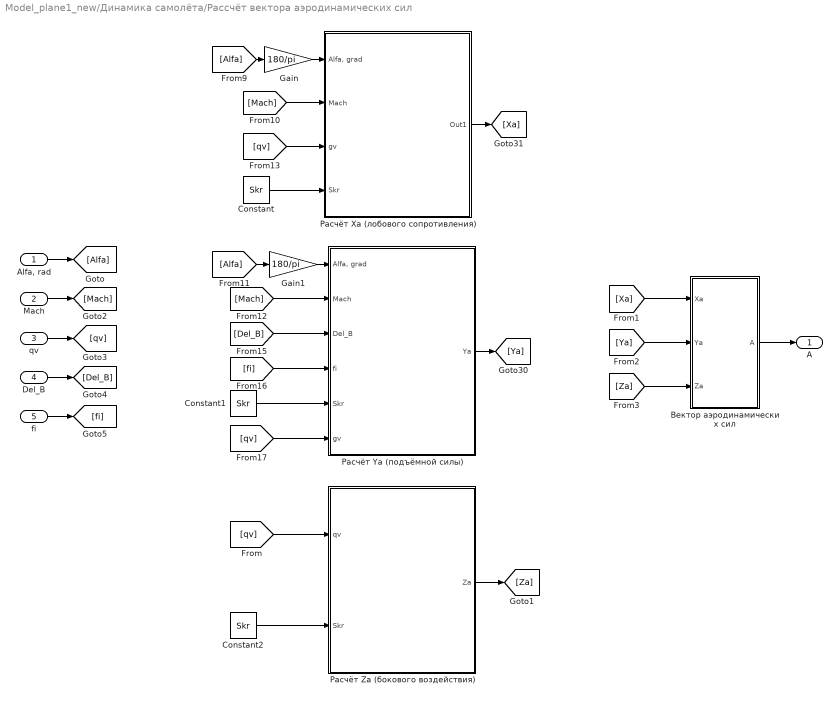
== system Model_plane1_new/Динамика самолёта/Рассчёт вектора аэродинамических сил ==
  "Alfa, rad" : Inport
  Mach : Inport  Port=2
  qv : Inport  Port=3
  Del_B : Inport  Port=4
  fi : Inport  Port=5
  Constant : Constant  Value=Skr
  Constant1 : Constant  Value=Skr
  Constant2 : Constant  Value=Skr
  Gain : Gain  Gain=180/pi
  Gain1 : Gain  Gain=180/pi
  Вектор аэродинамических сил : MATLAB Function  TreatAsAtomicUnit=on
  Расчёт Xa (лобового сопротивления) : Subsystem
  Расчёт Ya (подъёмной силы) : Subsystem
  Расчёт Za (бокового воздействия) : Subsystem
  A : Outport
  wires:
  Constant1/1 -> Расчёт Ya (подъёмной силы)/5(Skr)
  [qv] -> Расчёт Ya (подъёмной силы)/6(gv)
  Расчёт Ya (подъёмной силы)/1(Ya) -> [Ya]
  [Mach] -> Расчёт Xa (лобового сопротивления)/2(Mach)
  [Mach] -> Расчёт Ya (подъёмной силы)/2(Mach)
  [fi] -> Расчёт Ya (подъёмной силы)/4(fi)
  Расчёт Xa (лобового сопротивления)/1(Out1) -> [Xa]
  [qv] -> Расчёт Xa (лобового сопротивления)/3(gv)
  [Del_B] -> Расчёт Ya (подъёмной силы)/3(Del_B)
  Расчёт Za (бокового воздействия)/1(Za) -> [Za]
  "Alfa, rad"/1 -> [Alfa]
  Mach/1 -> [Mach]
  qv/1 -> [qv]
  Constant/1 -> Расчёт Xa (лобового сопротивления)/4(Skr)
  Del_B/1 -> [Del_B]
  fi/1 -> [fi]
  [qv] -> Расчёт Za (бокового воздействия)/1(qv)
  Constant2/1 -> Расчёт Za (бокового воздействия)/2(Skr)
  [Xa] -> Вектор аэродинамических сил/1(Xa)
  [Ya] -> Вектор аэродинамических сил/2(Ya)
  [Za] -> Вектор аэродинамических сил/3(Za)
  Вектор аэродинамических сил/1(A) -> A/1
  [Alfa] -> Gain1/1
  Gain1/1 -> Расчёт Ya (подъёмной силы)/1("Alfa, grad")
  Gain/1 -> Расчёт Xa (лобового сопротивления)/1("Alfa, grad")
  [Alfa] -> Gain/1

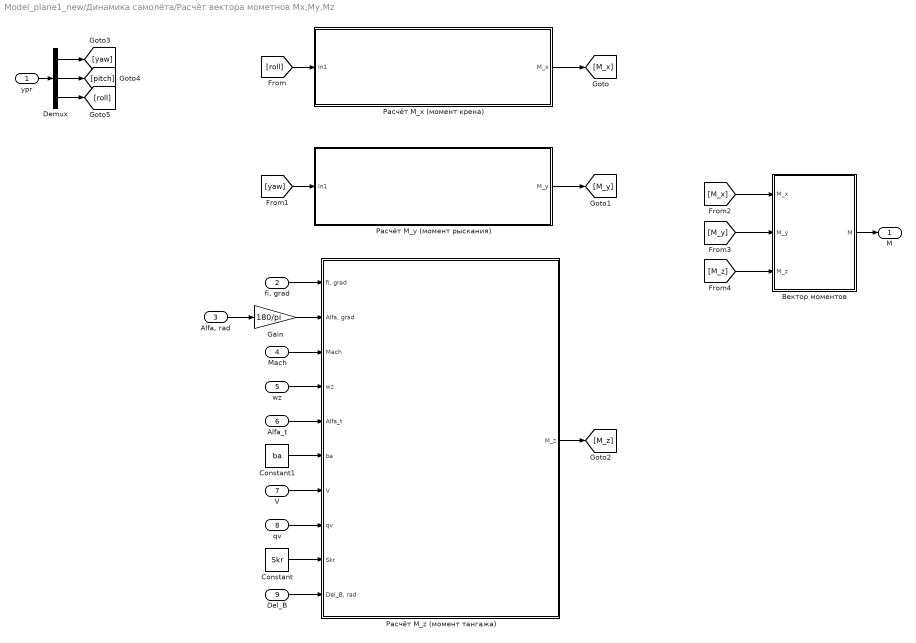
== system Model_plane1_new/Динамика самолёта/Расчёт вектора мометнов Mx,My,Mz ==
  ypr : Inport
  "fi, grad" : Inport  Port=2
  "Alfa, rad" : Inport  Port=3
  Mach : Inport  Port=4
  wz : Inport  Port=5
  Alfa_t : Inport  Port=6
  V : Inport  Port=7
  qv : Inport  Port=8
  Del_B : Inport  Port=9
  Constant : Constant  Value=Skr
  Constant1 : Constant  Value=ba
  Demux : Demux  Outputs=3
  Gain : Gain  Gain=180/pi
  Вектор моментов : MATLAB Function  TreatAsAtomicUnit=on
  Расчёт M_x (момент крена) : Subsystem
  Расчёт M_y (момент рыскания) : Subsystem
  Расчёт M_z (момент тангажа) : Subsystem
  M : Outport
  wires:
  Alfa_t/1 -> Расчёт M_z (момент тангажа)/5(Alfa_t)
  Del_B/1 -> Расчёт M_z (момент тангажа)/10("Del_B, rad")
  "Alfa, rad"/1 -> Gain/1
  qv/1 -> Расчёт M_z (момент тангажа)/8(qv)
  Расчёт M_z (момент тангажа)/1(M_z) -> [M_z]
  Constant/1 -> Расчёт M_z (момент тангажа)/9(Skr)
  V/1 -> Расчёт M_z (момент тангажа)/7(V)
  Mach/1 -> Расчёт M_z (момент тангажа)/3(Mach)
  wz/1 -> Расчёт M_z (момент тангажа)/4(wz)
  "fi, grad"/1 -> Расчёт M_z (момент тангажа)/1("fi, grad")
  Constant1/1 -> Расчёт M_z (момент тангажа)/6(ba)
  Расчёт M_x (момент крена)/1(M_x) -> [M_x]
  Расчёт M_y (момент рыскания)/1(M_y) -> [M_y]
  [roll] -> Расчёт M_x (момент крена)/1(In1)
  [yaw] -> Расчёт M_y (момент рыскания)/1(In1)
  [M_x] -> Вектор моментов/1(M_x)
  [M_y] -> Вектор моментов/2(M_y)
  [M_z] -> Вектор моментов/3(M_z)
  Вектор моментов/1(M) -> M/1
  ypr/1 -> Demux/1
  Demux/1 -> [yaw]
  Demux/2 -> [pitch]
  Demux/3 -> [roll]
  Gain/1 -> Расчёт M_z (момент тангажа)/2("Alfa, grad")

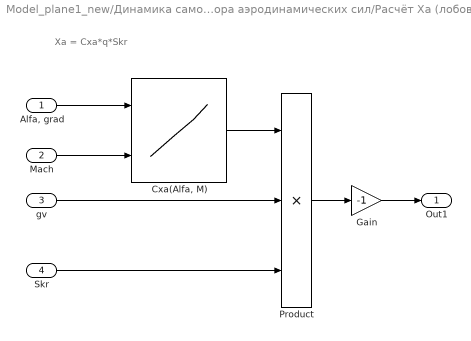
== system Model_plane1_new/Динамика самолёта/Рассчёт вектора аэродинамических сил/Расчёт Xa (лобового сопротивления) ==
  note: Xa = Cxa*q*Skr
  "Alfa, grad" : Inport
  Mach : Inport  Port=2
  gv : Inport  Port=3
  Skr : Inport  Port=4
  "Cxa(Alfa, M)" : Lookup_n-D  BreakpointsForDimension1=Alfa_table  BreakpointsForDimension2=M_table  Table=Cxa_table  InternalRulePriority=Speed  RndMeth=Simplest
      settings: InputPortMap=u0,u1
  Gain : Gain  Gain=-1
  Product : Product  Inputs=3
  Out1 : Outport
  wires:
  "Alfa, grad"/1 -> "Cxa(Alfa, M)"/1
  Skr/1 -> Product/3
  gv/1 -> Product/2
  Mach/1 -> "Cxa(Alfa, M)"/2
  "Cxa(Alfa, M)"/1 -> Product/1
  Product/1 -> Gain/1
  Gain/1 -> Out1/1

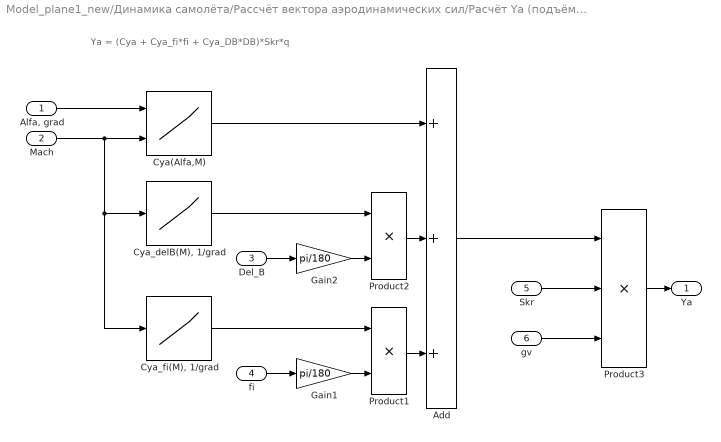
== system Model_plane1_new/Динамика самолёта/Рассчёт вектора аэродинамических сил/Расчёт Ya (подъёмной силы) ==
  note: Ya = (Cya + Cya_fi*fi + Cya_DB*DB)*Skr*q
  "Alfa, grad" : Inport
  Mach : Inport  Port=2
  Del_B : Inport  Port=3
  fi : Inport  Port=4
  Skr : Inport  Port=5
  gv : Inport  Port=6
  Add : Sum  Inputs=+++
  Cya(Alfa,M) : Lookup_n-D  BreakpointsForDimension1=Alfa_y  BreakpointsForDimension2=M_y  Table=Cya  InternalRulePriority=Speed  RndMeth=Simplest
      settings: InputPortMap=u0,u1
  "Cya_delB(M), 1/grad" : Lookup_n-D  NumberOfTableDimensions=1  BreakpointsForDimension1=M_C  Table=Cy_DB  InternalRulePriority=Speed  RndMeth=Simplest
  "Cya_fi(M), 1/grad" : Lookup_n-D  NumberOfTableDimensions=1  BreakpointsForDimension1=M_C  Table=Cy_fi  InternalRulePriority=Speed  RndMeth=Simplest
  Gain1 : Gain  Gain=pi/180
  Gain2 : Gain  Gain=pi/180
  Product1 : Product
  Product2 : Product
  Product3 : Product  Inputs=3
  Ya : Outport
  wires:
  "Alfa, grad"/1 -> Cya(Alfa,M)/1
  gv/1 -> Product3/3
  Skr/1 -> Product3/2
  Product3/1 -> Ya/1
  "Cya_fi(M), 1/grad"/1 -> Product1/1
  "Cya_delB(M), 1/grad"/1 -> Product2/1
  Mach/1 -> "Cya_delB(M), 1/grad"/1, "Cya_fi(M), 1/grad"/1, Cya(Alfa,M)/2
  Cya(Alfa,M)/1 -> Add/1
  Product2/1 -> Add/2
  Product1/1 -> Add/3
  Add/1 -> Product3/1
  Gain2/1 -> Product2/2
  fi/1 -> Gain1/1
  Gain1/1 -> Product1/2
  Del_B/1 -> Gain2/1

== system Model_plane1_new/Динамика самолёта/Рассчёт вектора аэродинамических сил/Расчёт Za (бокового воздействия) ==
  note: Za = Cza*q*Skr
  qv : Inport
  Skr : Inport  Port=2
  MATLAB Function : MATLAB Function  TreatAsAtomicUnit=on
  Za : Outport
  wires:
  qv/1 -> MATLAB Function/1(qv)
  Skr/1 -> MATLAB Function/2(Skr)
  MATLAB Function/1(Za) -> Za/1

== system Model_plane1_new/Динамика самолёта/Расчёт вектора мометнов Mx,My,Mz/Расчёт M_x (момент крена) ==
  In1 : Inport
  MATLAB Function : MATLAB Function  TreatAsAtomicUnit=on
  M_x : Outport
  wires:
  In1/1 -> MATLAB Function/1(u)
  MATLAB Function/1(M_x) -> M_x/1

== system Model_plane1_new/Динамика самолёта/Расчёт вектора мометнов Mx,My,Mz/Расчёт M_y (момент рыскания) ==
  In1 : Inport
  MATLAB Function : MATLAB Function  TreatAsAtomicUnit=on
  M_y : Outport
  wires:
  In1/1 -> MATLAB Function/1(u)
  MATLAB Function/1(M_y) -> M_y/1

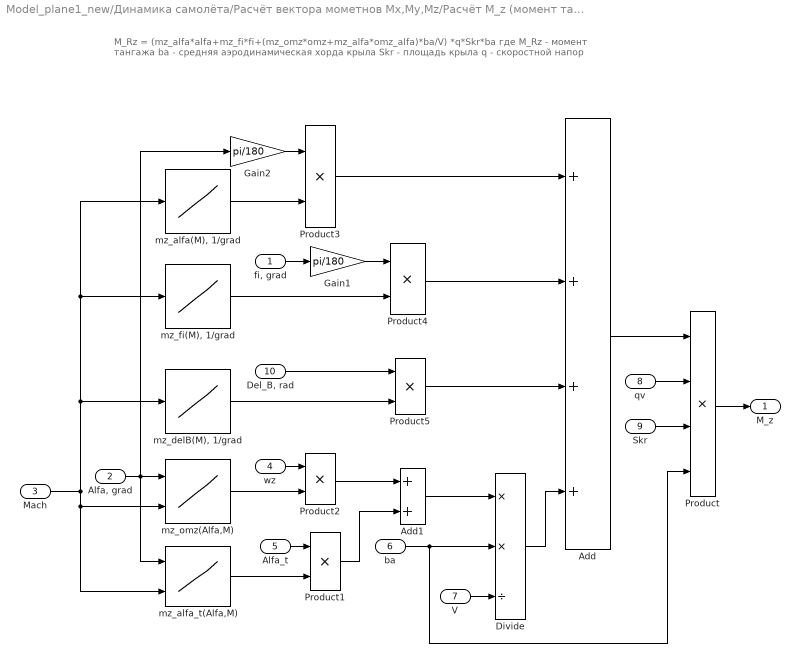
== system Model_plane1_new/Динамика самолёта/Расчёт вектора мометнов Mx,My,Mz/Расчёт M_z (момент тангажа) ==
  note: M_Rz = (mz_alfa*alfa+mz_fi*fi+(mz_omz*omz+mz_alfa*omz_alfa)*ba/V) *q*Skr*ba
      | где M_Rz - момент тангажа
      | ba - средняя аэродинамическая хорда крыла
      | Skr - площадь крыла
      | q - скоростной напор
  "fi, grad" : Inport
  "Alfa, grad" : Inport  Port=2
  Mach : Inport  Port=3
  wz : Inport  Port=4
  Alfa_t : Inport  Port=5
  ba : Inport  Port=6
  V : Inport  Port=7
  qv : Inport  Port=8
  Skr : Inport  Port=9
  "Del_B, rad" : Inport  Port=10
  Add : Sum  Inputs=++++
  Add1 : Sum
  Divide : Product  Inputs=**/
  Gain1 : Gain  Gain=pi/180
  Gain2 : Gain  Gain=pi/180
  Product : Product  Inputs=4
  Product{1..5} (5 alike) : Product
  "mz_alfa(M), 1/grad" : Lookup_n-D  NumberOfTableDimensions=1  BreakpointsForDimension1=M_mz  Table=mz_alfa  InternalRulePriority=Speed  RndMeth=Simplest
  mz_alfa_t(Alfa,M) : Lookup_n-D  BreakpointsForDimension1=Alfa  BreakpointsForDimension2=M_mz2  Table=mz_alfa2  InternalRulePriority=Speed  RndMeth=Simplest
      settings: InputPortMap=u0,u1
  "mz_delB(M), 1/grad" : Lookup_n-D  NumberOfTableDimensions=1  BreakpointsForDimension1=M_mz  Table=mz_DB  InternalRulePriority=Speed  RndMeth=Simplest
  "mz_fi(M), 1/grad" : Lookup_n-D  NumberOfTableDimensions=1  BreakpointsForDimension1=M_mz  Table=mz_fi  InternalRulePriority=Speed  RndMeth=Simplest
  mz_omz(Alfa,M) : Lookup_n-D  BreakpointsForDimension1=Alfa  BreakpointsForDimension2=M_mz2  Table=mz_omz  InternalRulePriority=Speed  RndMeth=Simplest
      settings: InputPortMap=u0,u1
  M_z : Outport
  wires:
  Product/1 -> M_z/1
  ba/1 -> Product/4, Divide/2
  Skr/1 -> Product/3
  qv/1 -> Product/2
  Add/1 -> Product/1
  V/1 -> Divide/3
  Divide/1 -> Add/4
  Add1/1 -> Divide/1
  Product2/1 -> Add1/1
  Product1/1 -> Add1/2
  Alfa_t/1 -> Product1/1
  wz/1 -> Product2/1
  mz_omz(Alfa,M)/1 -> Product2/2
  mz_alfa_t(Alfa,M)/1 -> Product1/2
  Mach/1 -> mz_omz(Alfa,M)/2, mz_alfa_t(Alfa,M)/2, "mz_alfa(M), 1/grad"/1, "mz_fi(M), 1/grad"/1, "mz_delB(M), 1/grad"/1
  "mz_alfa(M), 1/grad"/1 -> Product3/2
  "mz_fi(M), 1/grad"/1 -> Product4/2
  Product3/1 -> Add/1
  Product4/1 -> Add/2
  Product5/1 -> Add/3
  "Del_B, rad"/1 -> Product5/1
  "fi, grad"/1 -> Gain1/1
  Gain1/1 -> Product4/1
  "Alfa, grad"/1 -> Gain2/1, mz_omz(Alfa,M)/1, mz_alfa_t(Alfa,M)/1
  Gain2/1 -> Product3/1
  "mz_delB(M), 1/grad"/1 -> Product5/2

== matlab function Model_plane1_new/Динамика самолёта/Вектор состояния/Расчёт скорости ==
  data: Fkx input; dV output; mla input
function dV = fcn(Fkx, mla)

dV=Fkx/mla;

== matlab function Model_plane1_new/Динамика самолёта/Вектор состояния/Рассчёт скоростей в земной СК ==
  data: V input; dx output; Teta input; Psi input; dy output; dz output
function [dx, dy, dz] = fcn(V, Teta, Psi)

dx=V*cos(Psi)*cos(Teta);
dy=V*sin(Teta);
dz=-V*sin(Psi)*cos(Teta);

== matlab function Model_plane1_new/Динамика самолёта/Вектор состояния/Рассчёт углового измнения момента wx ==
  data: Mx input; dwx output; I input; wy input; wz input
function dwx = fcn(Mx,I,wy,wz)

dwx=(Mx-(I(3)-I(2))*wy*wz)/I(1);

== matlab function Model_plane1_new/Динамика самолёта/Вектор состояния/Рассчёт изменения угла рыскания ==
  data: dyaw output; wy input; wz input; pitch input; roll input
function dyaw = fcn(wy,wz,pitch,roll)

dyaw=(wy*cos(roll)-wz*sin(roll))/cos(pitch);

== matlab function Model_plane1_new/Динамика самолёта/Вектор состояния/Вектор состояния ==
  data: dV input; S output; dTeta input; dPsi input; dxg input; dyg input; dzg input; dwx input; dwy input; dwz input; dyaw input; dpitch input; droll input
function S = fcn(dV,dTeta,dPsi,dxg,dyg,dzg,dwx,dwy,dwz,dyaw,dpitch,droll)

S=[dV;dTeta;dPsi;dxg;dyg;dzg;dwx;dwy;dwz;dyaw;dpitch;droll];

== matlab function Model_plane1_new/Динамика самолёта/Вектор состояния/Координаты положения в пространстве ==
  data: xg input; xyz output; yg input; zg input
function xyz = fcn(xg,yg,zg)

xyz=[xg;yg;zg];

== matlab function Model_plane1_new/Динамика самолёта/Вектор состояния/Вектор угловых скоростей ==
  data: wx input; w output; wy input; wz input
function w = fcn(wx,wy,wz)

w=[wx;wy;wz];

== matlab function Model_plane1_new/Динамика самолёта/Рассчёт вектора аэродинамических сил/Вектор аэродинамических сил ==
  data: Xa input; A output; Ya input; Za input
function A = fcn(Xa, Ya, Za)

A=[Xa;Ya;Za];

== matlab function Model_plane1_new/Динамика самолёта/Вектор состояния/Углы положения в пространстве ==
  data: yaw input; ypr output; pitch input; roll input
function ypr = fcn(yaw,pitch,roll)

ypr=[yaw;pitch;roll];

== matlab function Model_plane1_new/Динамика самолёта/Вектор состояния/Вектор V, Teta, Psi ==
  data: V input; VTP output; Teta input; Psi input
function VTP = fcn(V,Teta,Psi)

VTP=[V;Teta;Psi];

== matlab function Model_plane1_new/Динамика самолёта/Вектор состояния/MATLAB Function1 ==
  data: Teta input; Alfa output; pitch input; yaw input; Psi input; Beta output; roll input
function [Alfa, Beta] = fcn(Teta, pitch, yaw, Psi,roll)
%Alfa=pitch-Teta;
%Beta=yaw-Psi;

Alfa=-atan((sin(roll)*cos(Teta)*sin(yaw-Psi)-cos(roll)*sin(pitch)*cos(Teta)*cos(yaw-Psi)+cos(roll)*cos(pitch)*sin(Teta))/(cos(pitch)*cos(Teta)*cos(yaw-Psi)+sin(pitch)*sin(Teta)));
Beta=asin(cos(roll)*cos(Teta)*sin(yaw-Psi)+sin(roll)*sin(pitch)*cos(Teta)*cos(yaw-Psi)-sin(roll)*cos(pitch)*sin(Teta));

== matlab function Model_plane1_new/Динамика самолёта/Вектор состояния/Рассчёт угла наклона траектории ==
  data: Fky input; dTeta output; V input; mla input
function dTeta = fcn(Fky,V,mla)

dTeta=Fky/(mla*V);

== matlab function Model_plane1_new/Динамика самолёта/Вектор состояния/Расчёт угла пути ==
  data: Fkz input; dPsi output; mla input; V input; Teta input
function dPsi = fcn(Fkz,mla,V,Teta)
dPsi=-Fkz/(mla*V*cos(Teta));

== matlab function Model_plane1_new/Динамика самолёта/Вектор состояния/Рассчёт углового измнения момента wy ==
  data: My input; I input; wx input; wz input; dwy output
function dwy = fcn(My,I,wx,wz)

dwy=(My-(I(1)-I(2))*wx*wz)/I(2);

== matlab function Model_plane1_new/Динамика самолёта/Вектор состояния/Рассчёт углового измнения момента wz ==
  data: Mz input; I input; wx input; wy input; dwz output
function dwz = fcn(Mz,I,wx,wy)

dwz=(Mz-(I(2)-I(1))*wx*wy)/I(3);

== matlab function Model_plane1_new/Динамика самолёта/Вектор состояния/Рассчёт изменения угла тангажа ==
  data: wy input; wz input; roll input; dpitch output
function dpitch = fcn(wy,wz,roll)

dpitch=wy*sin(roll)+wz*cos(roll);

== matlab function Model_plane1_new/Динамика самолёта/Вектор состояния/Рассчёт изменения угла крена ==
  data: wx input; wy input; wz input; pitch input; roll input; droll output
function droll = fcn(wx,wy,wz,pitch,roll)

droll=wx-(wy*cos(roll)-wz*sin(roll))*tan(pitch);

== matlab function Model_plane1_new/Динамика самолёта/Расчёт вектора мометнов Mx,My,Mz/Расчёт M_y (момент рыскания)/MATLAB Function ==
  data: u input; M_y output
function M_y = fcn(u)
c=0;

M_y = c*u;

== matlab function Model_plane1_new/Динамика самолёта/Рассчёт вектора аэродинамических сил/Расчёт Za (бокового воздействия)/MATLAB Function ==
  data: qv input; Za output; Skr input
function Za = fcn(qv,Skr)
Cz=0;

Za=Cz*qv*Skr;

== matlab function Model_plane1_new/Динамика самолёта/Вектор состояния/MATLAB Function2 ==
  data: pitch input; roll_a output; Alfa input; roll input; Teta input; Beta input
function roll_a = fcn(pitch,Alfa,roll,Teta,Beta)

roll_a=asin((sin(pitch)*cos(Alfa)*sin(Beta)-cos(roll)*cos(pitch)*sin(Alfa)*sin(Beta)+sin(roll)*cos(pitch)*cos(Beta))/cos(Teta));

== matlab function Model_plane1_new/Динамика самолёта/Вектор состояния/MATLAB Function3 ==
  data: V input; Vx output; Alfa input
function Vx = fcn(V,Alfa)

Vx=sqrt(V^2/(1+(tan(-Alfa))^2));

== matlab function Model_plane1_new/Контур управления скоростью/MATLAB Function ==
  data: V_e input; u output; int_V_e input; dif_V_e input
function u = fcn(V_e, int_V_e, dif_V_e)
Kp = 0.9;
Ki = 0.009;
Kd = 0.09;

u = Kp*V_e + Ki*int_V_e+Kd*dif_V_e;
end

== matlab function Model_plane1_new/Динамика самолёта/MATLAB Function ==
  data: V input; U output; y input; dy input; pitch input; w_z input
function U = fcn(V,y,dy,pitch,w_z)

U=[V,y,dy,pitch,w_z];

== matlab function Model_plane1_new/Контур управления скоростью1/MATLAB Function ==
  data: H_e input; u output; int_H_e input; dif_H_e input
function u = fcn(H_e, int_H_e, dif_H_e)
Kp = 0.01;
Ki = 0.000003;
Kd = 0.0009;

u = Kp*H_e + Ki*int_H_e+Kd*dif_H_e;
end

== matlab function Model_plane1_new/Динамика самолёта/Вектор тяги двигателя/Вектор тяги ==
  data: Px input; P output; Py input
function P = fcn(Px,Py)

P=[Px;Py;0];

== matlab function Model_plane1_new/Динамика самолёта/Вектор внешних сил/MATLAB Function ==
  data: mla input; W output; g input
function W = fcn(mla,g)

W=[0;-mla*g;0];

== matlab function Model_plane1_new/Динамика самолёта/Вектор проекций аэродинамических сил/MATLAB Function ==
  data: A input; Fk output; P input; W input; Teta input; Psi input; Alfa input; Beta input; roll_a input; yaw input; pitch input; roll input
function Fk = fcn(A,P,W,Teta,Psi,Alfa,Beta,roll_a,yaw,pitch,roll)

yaw_a=Psi;
pitch_a=Teta;


D_g_k = [cos(Psi)*cos(Teta), sin(Teta), -sin(Psi)*cos(Teta);
        -cos(Psi)*sin(Teta), cos(Teta), sin(Psi)*sin(Teta);
        sin(Psi), 0, cos(Psi)];

D_gv = [cos(yaw_a)*cos(pitch_a), sin(pitch_a), -sin(yaw_a)*cos(pitch_a);
        -cos(yaw_a)*sin(pitch_a)*cos(roll_a) + sin(yaw_a)*sin(roll_a), cos(pitch_a)*cos(roll_a), cos(yaw_a)*sin(roll_a) + sin(yaw_a)*sin(pitch_a)*cos(roll_a);
        cos(yaw_a)*sin(pitch_a)*sin(roll_a) + sin(yaw_a)*cos(roll_a), -cos(pitch_a)*sin(roll_a), cos(yaw_a)*cos(roll_a) - sin(yaw_a)*sin(pitch_a)*sin(roll_a)];
 
D_g_cv=[cos(yaw)*cos(pitch), sin(pitch), -sin(yaw)*cos(pitch);
    sin(yaw)*sin(roll)-cos(yaw)*sin(pitch)*cos(roll), cos(pitch)*cos(roll), cos(yaw)*sin(roll)+sin(yaw)*sin(pitch)*cos(roll);
    sin(yaw)*cos(roll)+cos(yaw)*sin(pitch)*sin(roll), -cos(pitch)*sin(roll), cos(yaw)*cos(roll)-sin(yaw)*sin(pitch)*sin(roll)];

D_cv_a = [cos(Alfa)*cos(Beta), -sin(Alfa)*cos(Beta), sin(Beta);
        sin(Alfa), cos(Alfa), 0;
        -cos(Alfa)*sin(Beta), sin(Alfa)*sin(Beta), cos(Beta)];

Fk = D_g_k * (D_g_cv' * (D_cv_a' * A + P) + W);

== matlab function Model_plane1_new/Динамика самолёта/Блок расчёта параметров стандартной атмосферы/MATLAB Function ==
  data: ro input; a input; q output; V input; M output
function [q, M] = fcn(ro, a, V)

q=(ro*V^2)/2;
M=V/a;

== matlab function Model_plane1_new/Динамика самолёта/Расчёт вектора мометнов Mx,My,Mz/Расчёт M_x (момент крена)/MATLAB Function ==
  data: u input; M_x output
function M_x = fcn(u)
c=0;

M_x = c*u;

== matlab function Model_plane1_new/Динамика самолёта/Вектор тяги двигателя/Проекции аэродинамических сил ==
  data: Px output; fi_p input; P input; alfa_Rud input; n_dvig input; Py output
function [Px, Py] = fcn(fi_p,P,alfa_Rud,n_dvig)

Px=cos(fi_p)*(n_dvig*alfa_Rud*P);
Py=sin(fi_p)*(n_dvig*alfa_Rud*P);

== matlab function Model_plane1_new/Динамика самолёта/Расчёт вектора мометнов Mx,My,Mz/Вектор моментов ==
  data: M_x input; M output; M_y input; M_z input
function M = fcn(M_x, M_y, M_z)

M=[M_x; M_y; M_z];
